simulink library "sc_toolbox"  (R2019a)
settings: Solver=VariableStepAuto  StartTime=0.0  StopTime=10.0  RelTol=1e-3
settings Model: Creator=mario  LastModifiedBy=mario

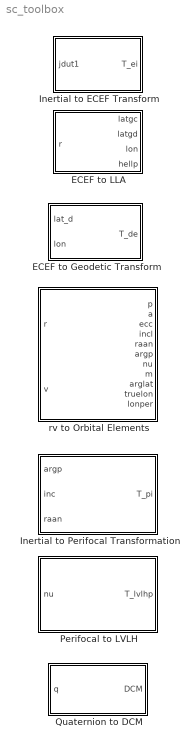
== system sc_toolbox ==
  ECEF to Geodetic Transform : MATLAB Function  TreatAsAtomicUnit=on
  ECEF to LLA : MATLAB Function  TreatAsAtomicUnit=on
  Inertial to ECEF Transform : MATLAB Function  TreatAsAtomicUnit=on
  Inertial to Perifocal Transformation : MATLAB Function  TreatAsAtomicUnit=on
  Perifocal to LVLH : MATLAB Function  TreatAsAtomicUnit=on
  Quaternion to DCM : MATLAB Function  TreatAsAtomicUnit=on
  rv to Orbital Elements : MATLAB Function  TreatAsAtomicUnit=on

== matlab function sc_toolbox/ECEF to LLA ==
  data: r input; latgc output; latgd output; lon output; hellp output
    %
    % ------------------------------------------------------------------------------
    %
    %                           function ecef2llb
    %
    %  these subroutines convert a geocentric equatorial (ijk) position vector into
    %    latitude and longitude.  geodetic and geocentric latitude are found.
    %
    %  author        : david vallado                  719-573-2600    9 jun 2002
    %
    %  revisions
    %                -
    %
    %  inputs          description                    range / units
    %    r           - ijk position vector            km
    %
    %  outputs       :
    %    latgc       - geocentric latitude            -pi to pi rad
    %    latgd       - geodetic latitude              -pi to pi rad
    %    lon         - longitude (west -)             -2pi to 2pi rad
    %    hellp       - height above the ellipsoid     km
    %
    %  locals        :
    %    rc          - range of site wrt earth center er
    %    height      - height above earth wrt site    er
    %    alpha       - angle from iaxis to point, lst rad
    %    olddelta    - previous value of deltalat     rad
    %    deltalat    - diff between delta and
    %                  geocentric lat                 rad
    %    delta       - declination angle of r in ijk  rad
    %    rsqrd       - magnitude of r squared         er2
    %    sintemp     - sine of temp                   rad
    %    c           -
    %
    %  coupling      :
    %    mag         - magnitude of a vector
    %    gcgd        - converts between geocentric and geodetic latitude
    %
    %  references    :
    %    vallado       2001, 174-179, alg 12 and alg 13, ex 3-3
    %
    % [latgc,latgd,lon,hellp] = ecef2llb ( r );
    % ------------------------------------------------------------------------------

    function [latgc,latgd,lon,hellp] = ecef2llb ( r )

    twopi =     2.0*pi;
    small =     0.00000001;

    % -------------------------  implementation   -------------------------
    % ---------------- find longitude value  ----------------------
    temp = sqrt( r(1)*r(1) + r(2)*r(2) );
    if ( abs( temp ) < small )
        rtasc= sign(r(3))*pi*0.5;
    else
        rtasc= atan2( r(2) , r(1) );
    end
    lon  = rtasc;
    if ( abs(lon) >= pi )
        if ( lon < 0.0  )
            lon= twopi + lon;
        else
            lon= lon - twopi;
        end
    end

    a= 6378.1363;
    % b = sign(r(3)) * 6356.75160056;
    b = sign(r(3)) * a * sqrt(1.0 - 0.006694385);  % find semiminor axis of the earth

    % -------------- set up initial latitude value  ---------------
    atemp= 1.0 /(a*temp);
    e= (b*r(3)-a*a+b*b)*atemp;
    f= (b*r(3)+a*a-b*b)*atemp;
    third= 1.0 /3.0;
    p= 4.0 *third*(e*f + 1.0  );
    q= 2.0 *(e*e - f*f);
    d= p*p*p + q*q;

    if ( d > 0.0  )
        nu= (sqrt(d)-q)^third - (sqrt(d)+q)^third;
    else
        sqrtp= sqrt(-p);
        nu= 2.0 *sqrtp*cos( third*acos(q/(p*sqrtp)) );
    end
    g= 0.5 *(sqrt(e*e + nu) + e);
    t= sqrt(g*g + (f-nu*g)/(2.0 *g-e)) - g;

    latgd= atan(a*(1.0 -t*t)/(2.0 *b*t));
    hellp= (temp-a*t)*cos( latgd) + (r(3)-b)*sin(latgd);

    latgc = asin(r(3)/norm(r));   % all locations
    %latgc = gd2gc(latgd);  % surface of the Earth locations

== matlab function sc_toolbox/Inertial to ECEF Transform ==
  data: jdut1 input; T_ei output
function T_ei = i2ecef(jdut1)

theta_gst = gstime(jdut1);

T_ei = [cos(theta_gst) sin(theta_gst) 0;
        -sin(theta_gst) cos(theta_gst) 0;
        0 0 1];

% -----------------------------------------------------------------------------
%
%                           function gstime
%
%  this function finds the greenwich sidereal time (iau-82).
%
%  author        : david vallado                  719-573-2600    7 jun 2002
%
%  revisions
%                -
%
%  inputs          description                    range / units
%    jdut1       - julian date of ut1             days from 4713 bc
%
%  outputs       :
%    gst         - greenwich sidereal time        0 to 2pi rad
%
%  locals        :
%    temp        - temporary variable for reals   rad
%    tut1        - julian centuries from the
%                  jan 1, 2000 12 h epoch (ut1)
%
%  coupling      :
%
%  references    :
%    vallado       2007, 193, Eq 3-43
%
% gst = gstime(jdut1);
% -----------------------------------------------------------------------------

function gst = gstime(jdut1)

        twopi      = 2.0*pi;
        deg2rad    = pi/180.0;

        % ------------------------  implementation   ------------------
        tut1= ( jdut1 - 2451545.0 ) / 36525.0;

        temp = - 6.2e-6 * tut1 * tut1 * tut1 + 0.093104 * tut1 * tut1  ...
               + (876600.0 * 3600.0 + 8640184.812866) * tut1 + 67310.54841;

        % 360/86400 = 1/240, to deg, to rad
        temp = rem( temp*deg2rad/240.0,twopi );

        % ------------------------ check quadrants --------------------
        if ( temp < 0.0 )
            temp = temp + twopi;
        end

        gst = temp;

== matlab function sc_toolbox/ECEF to Geodetic Transform ==
  data: lat_d input; T_de output; lon input
function T_de = ecef2d(lat_d,lon)

T_de = [-sin(lat_d)*cos(lon) -sin(lat_d)*sin(lon) cos(lat_d);
        -sin(lon) cos(lon) 0;
        -cos(lat_d)*cos(lon) -cos(lat_d)*sin(lon) -sin(lat_d)];

== matlab function sc_toolbox/rv to Orbital Elements ==
  data: r input; p output; v input; a output; ecc output; incl output; raan output; argp output; nu output; m output; arglat output; truelon output; lonper output
% ------------------------------------------------------------------------------
%
%                           function rv2coe
%
%  this function finds the classical orbital elements given the geocentric
%    equatorial position and velocity vectors.
%
%  author        : david vallado                  719-573-2600   21 jun 2002
%
%  revisions
%    vallado     - fix special cases                              5 sep 2002
%    vallado     - delete extra check in inclination code        16 oct 2002
%    vallado     - add constant file use                         29 jun 2003
%    vallado     - add mu                                         2 apr 2007
%
%  inputs          description                    range / units
%    r           - ijk position vector            km
%    v           - ijk velocity vector            km / s
%    mu          - gravitational parameter        km3 / s2
%
%  outputs       :
%    p           - semilatus rectum               km
%    a           - semimajor axis                 km
%    ecc         - eccentricity
%    incl        - inclination                    0.0  to pi rad
%    raan       - longitude of ascending node    0.0  to 2pi rad
%    argp        - argument of perigee            0.0  to 2pi rad
%    nu          - true anomaly                   0.0  to 2pi rad
%    m           - mean anomaly                   0.0  to 2pi rad
%    arglat      - argument of latitude      (ci) 0.0  to 2pi rad
%    truelon     - true longitude            (ce) 0.0  to 2pi rad
%    lonper      - longitude of periapsis    (ee) 0.0  to 2pi rad
%
%  locals        :
%    hbar        - angular momentum h vector      km2 / s
%    ebar        - eccentricity     e vector
%    nbar        - line of nodes    n vector
%    c1          - v**2 - u/r
%    rdotv       - r dot v
%    hk          - hk unit vector
%    sme         - specfic mechanical energy      km2 / s2
%    i           - index
%    e           - eccentric, parabolic,
%                  hyperbolic anomaly             rad
%    temp        - temporary variable
%    typeorbit   - type of orbit                  ee, ei, ce, ci
%
%  coupling      :
%    mag         - magnitude of a vector
%    angl        - find the angl between two vectors
%    newtonnu    - find the mean anomaly
%
%  references    :
%    vallado       2007, 121, alg 9, ex 2-5
%
% [p,a,ecc,incl,raan,argp,nu,m,arglat,truelon,lonper ] = rv2coe (r,v);
% ------------------------------------------------------------------------------

function [p,a,ecc,incl,raan,argp,nu,m,arglat,truelon,lonper ] = rv2coe (r,v)

        infinite  = 999999.9;
        undefined = 999999.1;

        % -------------------------  mathematical  --------------------
        rad    = 180.0 / pi;
        twopi  = 2.0 * pi;
        halfpi = pi * 0.5;

        % -------------------------  conversions  ---------------------
        ft2m    =    0.3048;
        nm2m    = 1852;
        re      = 6378.1363;         % km
        mu         = 398600.4415;      % km3/s2
        muin = mu; % this is the km version
        small=1e-12;
        
        % -------------------------  implementation   -----------------
        magr = norm( r );
        magv = norm( v );
        % ------------------  find h n and e vectors   ----------------
        [hbar] = cross( r,v );
        magh = norm( hbar );
        nbar = zeros(3,1);
        ebar = zeros(3,1);
        if ( magh >= 0.0 )
            nbar(1)= -hbar(2);
            nbar(2)=  hbar(1);
            nbar(3)=   0.0;
            magn = norm( nbar );
            c1 = magv*magv - muin /magr;
            rdotv= dot( r,v );
            for i= 1 : 3
                ebar(i)= (c1*r(i) - rdotv*v(i))/muin;
            end
            ecc = norm( ebar );

            % ------------  find a e and semi-latus rectum   ----------
            sme= ( magv*magv*0.5  ) - ( muin /magr );
            if ( abs( sme ) > small )
                a= -muin  / (2.0 *sme);
              else
                a= infinite;
            end
            p = magh*magh/muin;

            % -----------------  find inclination   -------------------
            hk= hbar(3)/magh;
            incl= acos( hk );

            % --------  determine type of orbit for later use  --------
            % ------ elliptical, parabolic, hyperbolic inclined -------
            typeorbit= 'ei';
            if ( ecc < small )
                % ----------------  circular equatorial ---------------
                if  (incl<small) || (abs(incl-pi)<small)
                    typeorbit= 'ce';
                  else
                    % --------------  circular inclined ---------------
                    typeorbit= 'ci';
                end
              else
                % - elliptical, parabolic, hyperbolic equatorial --
                if  (incl<small) || (abs(incl-pi)<small)
                    typeorbit= 'ee';
                end
            end

            % ----------  find right ascension of ascending node ------------
            if ( magn > small )
                temp= nbar(1) / magn;
                if ( abs(temp) > 1.0  )
                    temp= sign(temp);
                end
                raan= acos( temp );
                if ( nbar(2) < 0.0  )
                    raan= twopi - raan;
                end
              else
                raan= undefined;
            end

            % ---------------- find argument of perigee ---------------
            if (strcmp(typeorbit, 'ei') == 1)
                argp = angl( nbar,ebar);
                if ( ebar(3) < 0.0  )
                    argp= twopi - argp;
                end
              else
                argp= undefined;
            end

            % ------------  find true anomaly at epoch    -------------
            if ( typeorbit(1:1) == 'e' )
                nu =  angl( ebar,r);
                if ( rdotv < 0.0  )
                    nu= twopi - nu;
                end
              else
                nu= undefined;
            end

            % ----  find argument of latitude - circular inclined -----
            % -- find in general cases too
            if (strcmp(typeorbit, 'ci') == 1) || (strcmp(typeorbit, 'ei') == 1)
                arglat = angl( nbar,r );
                if ( r(3) < 0.0  )
                    arglat= twopi - arglat;
                end
                m = arglat;
              else
                arglat= undefined;
            end

            % -- find longitude of perigee - elliptical equatorial ----
            if  ( ecc>small ) && (strcmp(typeorbit, 'ee') == 1)
                temp= ebar(1)/ecc;
                if ( abs(temp) > 1.0  )
                    temp= sign(temp);
                end
                lonper= acos( temp );
                if ( ebar(2) < 0.0  )
                    lonper= twopi - lonper;
                end
                if ( incl > halfpi )
                    lonper= twopi - lonper;
                end
              else
                lonper= undefined;
            end

            % -------- find true longitude - circular equatorial ------
            if  ( magr>small ) && (strcmp(typeorbit, 'ce') == 1)
                temp= r(1)/magr;
                if ( abs(temp) > 1.0  )
                    temp= sign(temp);
                end
                truelon= acos( temp );
                if ( r(2) < 0.0  )
                    truelon= twopi - truelon;
                end
                if ( incl > halfpi )
                    truelon= twopi - truelon;
                end
                m = truelon;
              else
                truelon= undefined;
            end

            % ------------ find mean anomaly for all orbits -----------
           % if ( typeorbit(1:1) == 'e' )
                [e,m] = newtonnu(ecc,nu );
           % end

         else
           p    = undefined;
           a    = undefined;
           ecc  = undefined;
           incl = undefined;
           raan= undefined;
           argp = undefined;
           nu   = undefined;
           m    = undefined;
           arglat = undefined;
           truelon= undefined;
           lonper = undefined;
       end

== matlab function sc_toolbox/Inertial to Perifocal Transformation ==
  data: argp input; T_pi output; inc input; raan input
function T_pi = i2pqw(argp,inc,raan)

T_xi = [cos(raan) sin(raan) 0;
        -sin(raan) cos(raan) 0;
        0 0 1];

T_yx = [0 0 1;
        cos(inc) sin(inc) 0;
        -sin(inc) cos(inc) 0];

T_py = [cos(argp) sin(argp) 0;
        -sin(argp) cos(argp) 0;
        0 0 1];


T_pi = T_py*T_yx*T_xi;

== matlab function sc_toolbox/Perifocal to LVLH ==
  data: nu input; T_lvlhp output
function T_lvlhp = pqw2lvlh(nu)

T_lvlhp = [cos(nu) sin(nu) 0;
            -sin(nu) cos(nu) 0;
            0 0 1];

== matlab function sc_toolbox/Quaternion to DCM ==
  data: q input; DCM output
function DCM = q2dcm(q)
q1 = q(1);
qbar = [q(2);q(3);q(4)];
qtilde = [0 -qbar(3) qbar(2);qbar(3) 0 -qbar(1);-qbar(2) qbar(1) 0];

DCM = 2*(qbar*qbar') + (q1^2-qbar'*qbar)*eye(3) - 2*q1*qtilde;
